simulink model "Trial_Sim_Jonny"  (R2020b)
settings: Solver=VariableStepAuto  StartTime=0.0  StopTime=10.0  RelTol=1e-3
values from neighbouring files (symbols this model uses):
  A_AD = horzcat(A_i, A_ii)    [Trial_Script.m]
  A_kal = [0 0 0 1 0 0 ... (first row only)    [Trial_Script.m]
  B_AD = horzcat(B_i, B_ii)    [Trial_Script.m]
  B_kal = [0 0 0 0 0 0 ... (first row only)    [Trial_Script.m]
  C_AD = eye(6)    [Trial_Script.m]
  C_D = 0.6    [Trial_Script.m]
  C_kal = eye(6)    [Trial_Script.m]
  D_AD = zeros(6)    [Trial_Script.m]
  D_kal = zeros(6)    [Trial_Script.m]
  g = 9.81    [Trial_Script.m]
  I_inv = Inertia_inv    [Trial_Script.m]
  m = 300    [Trial_Script.m]
  pid_Mx = [pid_Mx.Kp, pid_Mx.Ki, pid_Mx.Kd]    [Trial_Script.m]
  pid_My = [pid_My.Kp, pid_My.Ki, pid_My.Kd]    [Trial_Script.m]
  pid_Mz = [pid_Mz.Kp, pid_Mz.Ki, pid_Mz.Kd]    [Trial_Script.m]
  r_0 = [0;0;0]    [Trial_Script.m]
  rho = 1.225    [Trial_Script.m]
  S = 1*1.8    (= 1.8)    [Trial_Script.m]
  T = 10.5    [Trial_Script.m]    (also in temp2.m = readtable('proparms.txt','Delimiter',' '))
  time_delay = 0.1    [Trial_Script.m]
  v_0 = [0;0;0]    [Trial_Script.m]
  w_0 = [0;0;0]    [Trial_Script.m]
undefined symbols (not defined in the file or in its folder): Continuous, Time
libraries: pid_lib x6, ctrlSharedLib x2, simulink x2, dspmtrx3 x1
settings Model: Creator=Jonathan van Zyl  LastModifiedBy=Jonathan van Zyl

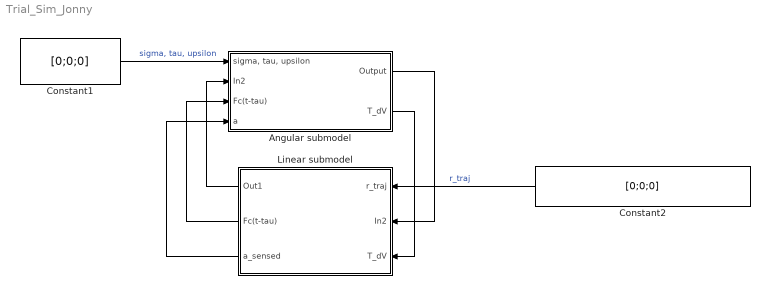
== system Trial_Sim_Jonny ==
  Angular submodel : Subsystem
  Constant1 : Constant  Value=[0;0;0]
  Constant2 : Constant  Value=[0;0;0]
  Linear submodel : Subsystem
  wires:
  Constant1/1 -> Angular submodel/1("sigma, tau, upsilon")  "sigma, tau, upsilon"
  Constant2/1 -> Linear submodel/1(r_traj)  "r_traj"
  Angular submodel/1(Output) -> Linear submodel/2(In2)
  Angular submodel/2(T_dV) -> Linear submodel/3(T_dV)
  Linear submodel/1(Out1) -> Angular submodel/2(In2)
  Linear submodel/2(Fc(t-tau)) -> Angular submodel/3(Fc(t-tau))
  Linear submodel/3(a_sensed) -> Angular submodel/4(a)

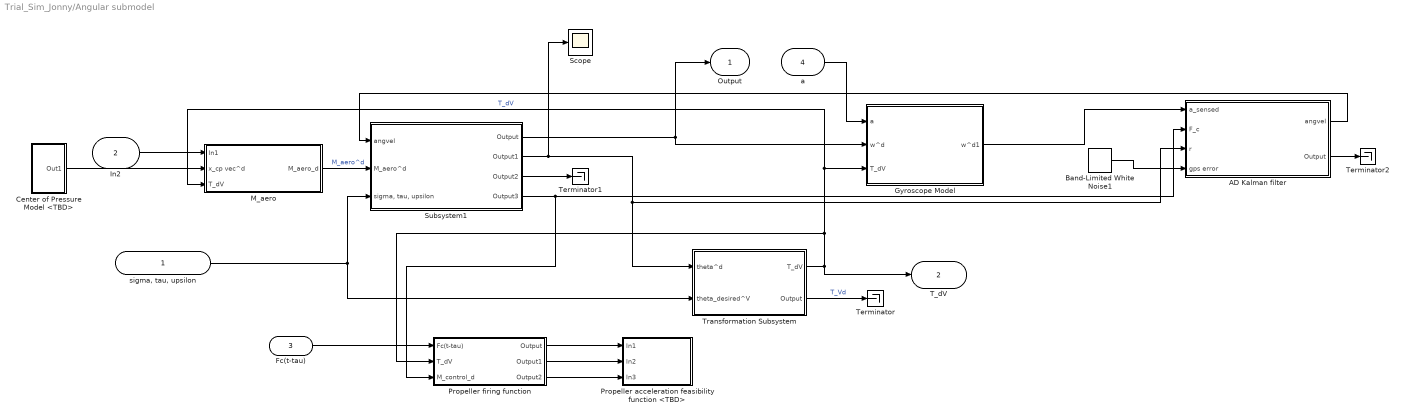
== system Trial_Sim_Jonny/Angular submodel ==
  "sigma, tau, upsilon" : Inport
  In2 : Inport  Port=2
  Fc(t-tau) : Inport  Port=3
  a : Inport  Port=4
  AD Kalman filter : Subsystem
  Band-Limited White Noise1 : simulink/Sources/Band-Limited White Noise  Cov=[0.00001]  Ts=0.1  seed=[23341]
  Center of Pressure Model <TBD> : Subsystem
  Gyroscope Model : Subsystem
  M_aero : Subsystem
  Propeller acceleration feasibility function <TBD> : Subsystem
  Propeller firing function : Subsystem
  Scope : Scope
  Subsystem1 : Subsystem
  Terminator : Terminator
  Terminator1 : Terminator
  Terminator2 : Terminator
  Transformation Subsystem : Subsystem
  Output : Outport
  T_dV : Outport  Port=2
  wires:
  Subsystem1/3(Output2) -> Terminator1/1
  Transformation Subsystem/1(T_dV) -> M_aero/3(T_dV), Gyroscope Model/3(T_dV), Propeller firing function/2(T_dV), T_dV/1  "T_dV"
  Subsystem1/4(Output3) -> Propeller firing function/3(M_control_d), AD Kalman filter/2(F_c)
  Propeller firing function/3(Output2) -> Propeller acceleration feasibility function <TBD>/3(In3)
  Center of Pressure Model <TBD>/1(Out1) -> M_aero/2(x_cp vec^d)
  "sigma, tau, upsilon"/1 -> Transformation Subsystem/2(theta_desired^V), Subsystem1/3("sigma, tau, upsilon")
  AD Kalman filter/1(angvel) -> Subsystem1/1(angvel)
  Propeller firing function/2(Output1) -> Propeller acceleration feasibility function <TBD>/2(In2)
  Subsystem1/2(Output1) -> Scope/1, AD Kalman filter/3(r), Transformation Subsystem/1(theta^d)
  M_aero/1(M_aero_d) -> Subsystem1/2(M_aero^d)  "M_aero^d"
  AD Kalman filter/2(Output) -> Terminator2/1
  Propeller firing function/1(Output) -> Propeller acceleration feasibility function <TBD>/1(In1)
  Transformation Subsystem/2(Output) -> Terminator/1  "T_Vd"
  Gyroscope Model/1(w^d1) -> AD Kalman filter/1(a_sensed)
  Subsystem1/1(Output) -> Output/1, Gyroscope Model/2(w^d)
  Band-Limited White Noise1/1 -> AD Kalman filter/4(gps error)
  a/1 -> Gyroscope Model/1(a)
  Fc(t-tau)/1 -> Propeller firing function/1(Fc(t-tau))
  In2/1 -> M_aero/1(In1)

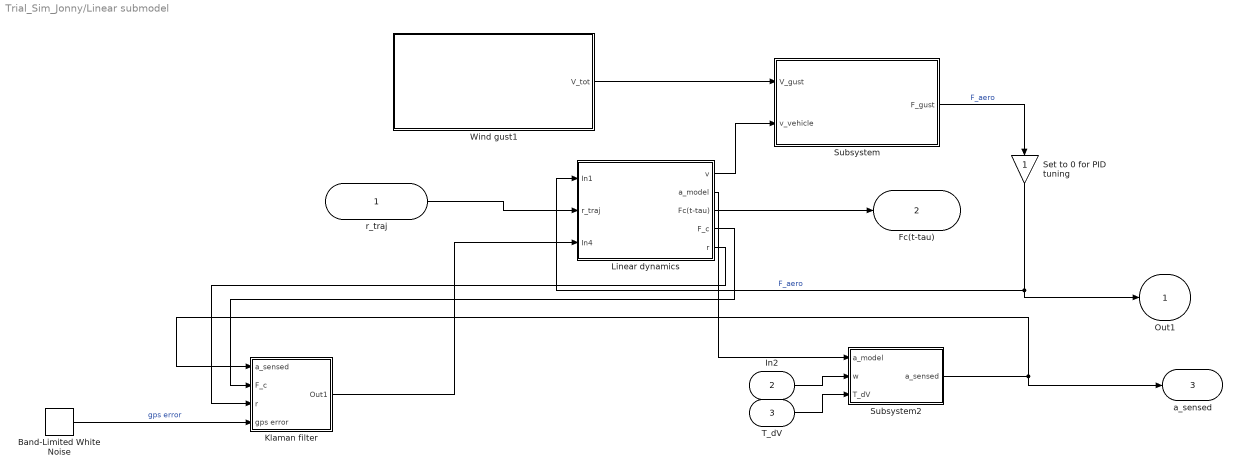
== system Trial_Sim_Jonny/Linear submodel ==
  r_traj : Inport
  In2 : Inport  Port=2
  T_dV : Inport  Port=3
  Band-Limited White Noise : simulink/Sources/Band-Limited White Noise  Cov=[0.00001]  Ts=0.1  seed=[23341]
  Klaman filter : Subsystem
  Linear dynamics : Subsystem
  Set to 0 for PID tuning : Gain
  Subsystem : Subsystem
  Subsystem2 : Subsystem
  Wind gust1 : Subsystem
  Out1 : Outport
  Fc(t-tau) : Outport  Port=2
  a_sensed : Outport  Port=3
  wires:
  Set to 0 for PID tuning/1 -> Out1/1, Linear dynamics/1(In1)  "F_aero"
  Linear dynamics/3(Fc(t-tau)) -> Fc(t-tau)/1
  Wind gust1/1(V_tot) -> Subsystem/1(V_gust)
  Band-Limited White Noise/1 -> Klaman filter/4(gps error)  "gps error"
  Subsystem2/1(a_sensed) -> Klaman filter/1(a_sensed), a_sensed/1
  Subsystem/1(F_gust) -> Set to 0 for PID tuning/1  "F_aero"
  Linear dynamics/1(v) -> Subsystem/2(v_vehicle)
  Klaman filter/1(Out1) -> Linear dynamics/3(In4)
  Linear dynamics/4(F_c) -> Klaman filter/2(F_c)
  Linear dynamics/5(r) -> Klaman filter/3(r)
  Linear dynamics/2(a_model) -> Subsystem2/1(a_model)
  In2/1 -> Subsystem2/2(w)
  T_dV/1 -> Subsystem2/3(T_dV)
  r_traj/1 -> Linear dynamics/2(r_traj)

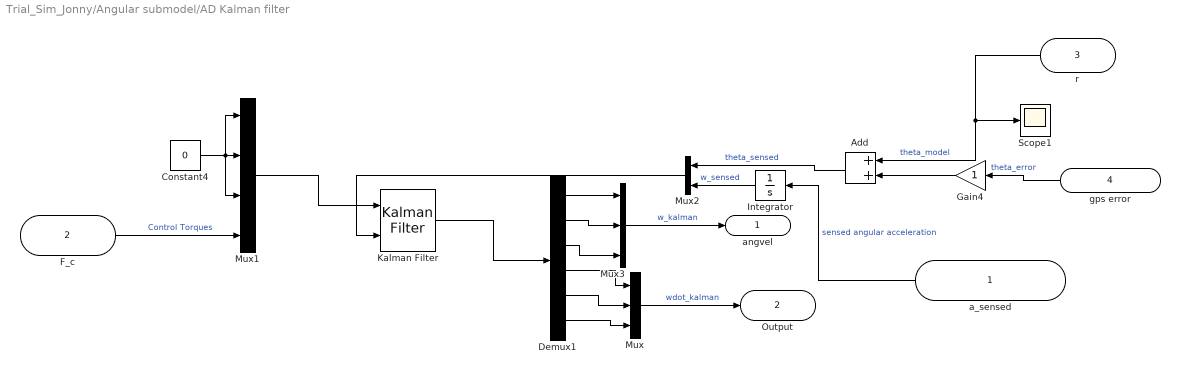
== system Trial_Sim_Jonny/Angular submodel/AD Kalman filter ==
  a_sensed : Inport
  F_c : Inport  Port=2
  r : Inport  Port=3
  gps error : Inport  Port=4
  Add : Sum
  Constant4 : Constant  Value=0
  Demux1 : Demux  Outputs=6
  Gain4 : Gain
  Integrator : Integrator  InitialCondition=w_0
  Kalman Filter : ctrlSharedLib/Kalman Filter  TimeDomain=Continuous-Time  UseCurrentEstimator=on  ModelSource=Individual A, B, C, D matrices  ModelSourceVariable=ss(0.95,1,1,0,1)  A=A_AD  B=B_AD  C=C_AD  D=D_AD  NumberOfStates=1  NumberOfInputs=1  NumberOfOutputs=1  InitialEstimateSource=Dialog  X0=[0;0;0;0;0;0]  P0=10  UseK=off  UseGH=off  NumberOfProcessNoiseInputs=1  G=1  TimeInvariantG=on  H=0  TimeInvariantH=on  Q=0.05  TimeInvariantQ=on  R=1  TimeInvariantR=on  N=0  TimeInvariantN=on  AddInputPort=on  AddEnablePort=off  OutputEstimatedY=off  OutputP=off  Ts=-1
  Mux : Mux  Inputs=3
  Mux1 : Mux
  Mux2 : Mux  Inputs=2
  Mux3 : Mux  Inputs=3
  Scope1 : Scope
  angvel : Outport
  Output : Outport  Port=2
  wires:
  Demux1/5 -> Mux/2
  Mux2/1 -> Kalman Filter/2
  Constant4/1 -> Mux1/3, Mux1/1, Mux1/2
  gps error/1 -> Gain4/1  "theta_error"
  r/1 -> Scope1/1, Add/1  "theta_model"
  Demux1/4 -> Mux/1
  Demux1/2 -> Mux3/2
  Mux1/1 -> Kalman Filter/1
  F_c/1 -> Mux1/4  "Control Torques"
  Demux1/1 -> Mux3/1
  Kalman Filter/1 -> Demux1/1
  Demux1/6 -> Mux/3
  Gain4/1 -> Add/2
  Demux1/3 -> Mux3/3
  Integrator/1 -> Mux2/2  "w_sensed"
  Add/1 -> Mux2/1  "theta_sensed"
  Mux3/1 -> angvel/1  "w_kalman"
  a_sensed/1 -> Integrator/1  "sensed angular acceleration"
  Mux/1 -> Output/1  "wdot_kalman"

== system Trial_Sim_Jonny/Angular submodel/Center of Pressure Model <TBD> ==
  Constant1 : Constant  Value=[0.1;0.2; 0.05]
  Out1 : Outport
  wires:
  Constant1/1 -> Out1/1  "x_cp"

== system Trial_Sim_Jonny/Angular submodel/Gyroscope Model ==
  a : Inport
  w^d : Inport  Port=2
  T_dV : Inport  Port=3
  Terminator : Terminator
  Terminator1 : Terminator
  w^d1 : Outport
  wires:
  w^d/1 -> w^d1/1
  T_dV/1 -> Terminator/1
  a/1 -> Terminator1/1

== system Trial_Sim_Jonny/Angular submodel/M_aero ==
  In1 : Inport
  x_cp vec^d : Inport  Port=2
  T_dV : Inport  Port=3
  Matrix Multiply : Product  Multiplication=Matrix(*)
  Matrix Multiply1 : Product
  M_aero_d : Outport
  wires:
  Matrix Multiply/1 -> Matrix Multiply1/2  "F_dis^d"
  x_cp vec^d/1 -> Matrix Multiply1/1  "x_cp"
  T_dV/1 -> Matrix Multiply/1
  In1/1 -> Matrix Multiply/2  "F_gust"
  Matrix Multiply1/1 -> M_aero_d/1  "M_aero_d"

== system Trial_Sim_Jonny/Angular submodel/Propeller acceleration feasibility function <TBD> ==
  In1 : Inport
  In2 : Inport  Port=2
  In3 : Inport  Port=3
  Terminator4 : Terminator
  Terminator5 : Terminator
  Terminator6 : Terminator
  wires:
  In1/1 -> Terminator4/1
  In2/1 -> Terminator5/1
  In3/1 -> Terminator6/1

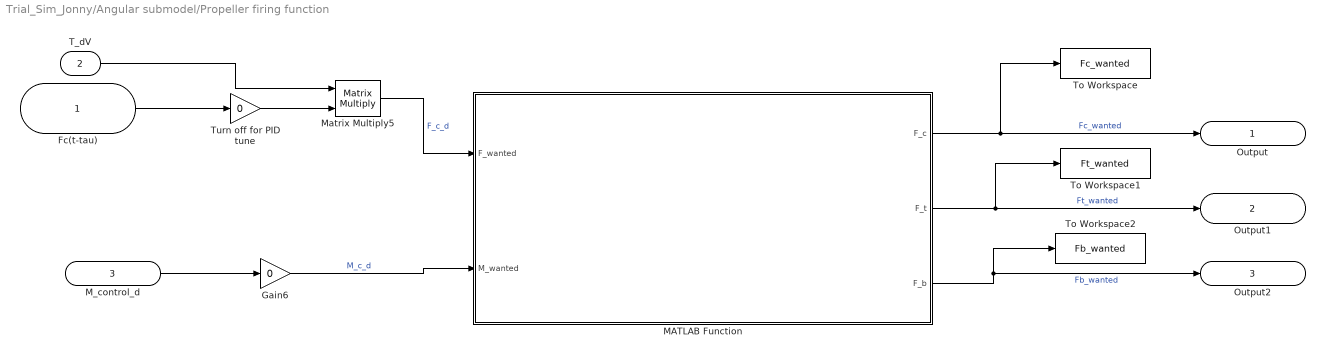
== system Trial_Sim_Jonny/Angular submodel/Propeller firing function ==
  Fc(t-tau) : Inport
  T_dV : Inport  Port=2
  M_control_d : Inport  Port=3
  Gain6 : Gain  Gain=0
  MATLAB Function : MATLAB Function  TreatAsAtomicUnit=on
  Matrix Multiply5 : Product  Multiplication=Matrix(*)
  To Workspace : ToWorkspace  VariableName=Fc_wanted  SaveFormat=Timeseries  SampleTime=-1
  To Workspace1 : ToWorkspace  VariableName=Ft_wanted  SaveFormat=Timeseries  SampleTime=-1
  To Workspace2 : ToWorkspace  VariableName=Fb_wanted  SaveFormat=Timeseries  SampleTime=-1
  Turn off for PID tune : Gain  Gain=0
  Output : Outport
  Output1 : Outport  Port=2
  Output2 : Outport  Port=3
  wires:
  Turn off for PID tune/1 -> Matrix Multiply5/2
  Fc(t-tau)/1 -> Turn off for PID tune/1
  Matrix Multiply5/1 -> MATLAB Function/1(F_wanted)  "F_c_d"
  T_dV/1 -> Matrix Multiply5/1
  M_control_d/1 -> Gain6/1
  Gain6/1 -> MATLAB Function/2(M_wanted)  "M_c_d"
  MATLAB Function/2(F_t) -> To Workspace1/1, Output1/1  "Ft_wanted"
  MATLAB Function/3(F_b) -> Output2/1, To Workspace2/1  "Fb_wanted"
  MATLAB Function/1(F_c) -> To Workspace/1, Output/1  "Fc_wanted"

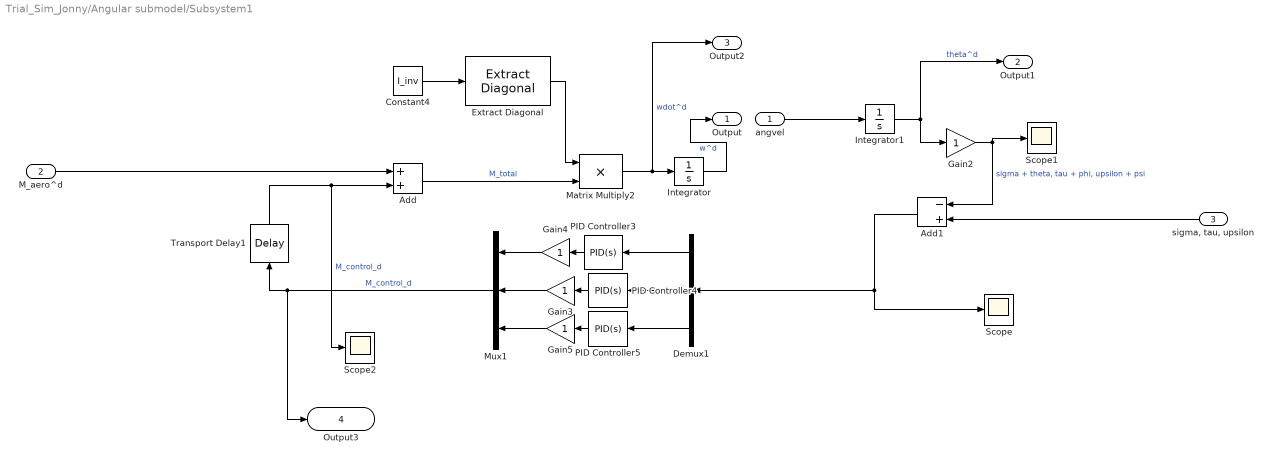
== system Trial_Sim_Jonny/Angular submodel/Subsystem1 ==
  angvel : Inport
  M_aero^d : Inport  Port=2
  "sigma, tau, upsilon" : Inport  Port=3
  Add : Sum
  Add1 : Sum  Inputs=-+
  Constant4 : Constant  Value=I_inv
  Demux1 : Demux  Outputs=3
  Extract Diagonal : dspmtrx3/Extract Diagonal
      settings: SourceProductBaseCode=DS
  Gain{2..5} (4 alike) : Gain
  Integrator : Integrator  InitialCondition=[0;0;0]
  Integrator1 : Integrator  InitialCondition=[0;0;0]
  Matrix Multiply2 : Product
  Mux1 : Mux  Inputs=3
  PID Controller3 : pid_lib/PID Controller  Controller=PID  Form=Parallel  TimeDomain=Continuous-time  UseExternalTs=off  SampleTime=-1  IntegratorMethod=Forward Euler  FilterMethod=Forward Euler  ControllerParametersSource=internal  P=pid_Mx(1)  I=pid_Mx(2)  D=pid_Mx(3)  UseFilter=on  N=546.991859681686  TunerSelectOption=Transfer Function Based (PID Tuner App)  InitialConditionSource=internal  InitialConditionForIntegrator=0  InitialConditionForFilter=0  DifferentiatorICPrevScaledInput=0  ExternalReset=none  TrackingMode=off  Kt=1  LimitOutput=off  SatLimitsSource=internal  UpperSaturationLimit=inf  LowerSaturationLimit=-inf  LinearizeAsGain=on  AntiWindupMode=none  Kb=1  POutMin=[]  POutMax=[]  IOutMin=[]  IOutMax=[]  DOutMin=[]  DOutMax=[]  NOutMin=[]  NOutMax=[]  SumOutMin=[]  SumOutMax=[]  SaturationOutMin=[]  SaturationOutMax=[]  PParamMin=[]  PParamMax=[]  IParamMin=[]  IParamMax=[]  DParamMin=[]  DParamMax=[]  NParamMin=[]  NParamMax=[]  KbParamMin=[]  KbParamMax=[]  KtParamMin=[]  KtParamMax=[]  KbOutMin=[]  KbOutMax=[]  KtOutMin=[]  KtOutMax=[]  IntegratorOutMin=[]  IntegratorOutMax=[]  FilterOutMin=[]  FilterOutMax=[]  SumI1OutMin=[]  SumI1OutMax=[]  SumI2OutMin=[]  SumI2OutMax=[]  SumI3OutMin=[]  SumI3OutMax=[]  SumI4OutMin=[]  SumI4OutMax=[]  SumDOutMin=[]  SumDOutMax=[]  DifferentiatorOutMin=[]  DifferentiatorOutMax=[]  FilterDiffOutCoefMin=[]  FilterDiffOutCoefMax=[]  ReciprocalOutMin=[]  ReciprocalOutMax=[]  SumDenOutMin=[]  SumDenOutMax=[]  SumNumOutMin=[]  SumNumOutMax=[]  DivideOutMin=[]  DivideOutMax=[]  UdiffTsProdOutMin=[]  UdiffTsProdOutMax=[]  NTsProdOutMin=[]  NTsProdOutMax=[]  UintegralTsProdOutMin=[]  UintegralTsProdOutMax=[]  UngainTsProdOutMin=[]  UngainTsProdOutMax=[]  IntegratorContinuousStateAttributes=''  IntegratorStateMustResolveToSignalObject=off  IntegratorRTWStateStorageClass=Auto  FilterContinuousStateAttributes=''  FilterStateMustResolveToSignalObject=off  FilterRTWStateStorageClass=Auto  ParallelPVariant=InternalParameters  IdealPVariant=Disabled  IVariant=InternalParameters  DVariant=InternalParameters  IntegratorVariant=Continuous  SatVariant=Disabled  AWVariant=Passthrough  PCopyVariant=Disabled  TRVariant=Disabled  FdbkBlocksVariant=Forward  IdealPFdbkVariant=Disabled  SatFdbkVariant=Disabled  DerivativeFilterVariant=ContFilter  NVariant=InternalParameters  NCopyVariant=Disabled  FilterICVariant=InternalICsFilter  IntegratorICVariant=InternalICs  ExternalResetVariant=Disabled  TRSumVariant=Passthrough  SumFdbkVariant=Disabled  SumVariant=Sum_PID  TsampFilterVariant=InternalTs  TsampNgainVariant=Passthrough  TsampIntegralVariant=Passthrough  ExternalSaturationOutDataTypeStr=Inherit: Same as second input
  PID Controller4 : pid_lib/PID Controller  Controller=PID  Form=Parallel  TimeDomain=Continuous-time  UseExternalTs=off  SampleTime=-1  IntegratorMethod=Forward Euler  FilterMethod=Forward Euler  ControllerParametersSource=internal  P=pid_My(1)  I=pid_My(2)  D=pid_My(3)  UseFilter=on  N=10.4897155810233  TunerSelectOption=Transfer Function Based (PID Tuner App)  InitialConditionSource=internal  InitialConditionForIntegrator=0  InitialConditionForFilter=0  DifferentiatorICPrevScaledInput=0  ExternalReset=none  TrackingMode=off  Kt=1  LimitOutput=off  SatLimitsSource=internal  UpperSaturationLimit=inf  LowerSaturationLimit=-inf  LinearizeAsGain=on  AntiWindupMode=none  Kb=1  POutMin=[]  POutMax=[]  IOutMin=[]  IOutMax=[]  DOutMin=[]  DOutMax=[]  NOutMin=[]  NOutMax=[]  SumOutMin=[]  SumOutMax=[]  SaturationOutMin=[]  SaturationOutMax=[]  PParamMin=[]  PParamMax=[]  IParamMin=[]  IParamMax=[]  DParamMin=[]  DParamMax=[]  NParamMin=[]  NParamMax=[]  KbParamMin=[]  KbParamMax=[]  KtParamMin=[]  KtParamMax=[]  KbOutMin=[]  KbOutMax=[]  KtOutMin=[]  KtOutMax=[]  IntegratorOutMin=[]  IntegratorOutMax=[]  FilterOutMin=[]  FilterOutMax=[]  SumI1OutMin=[]  SumI1OutMax=[]  SumI2OutMin=[]  SumI2OutMax=[]  SumI3OutMin=[]  SumI3OutMax=[]  SumI4OutMin=[]  SumI4OutMax=[]  SumDOutMin=[]  SumDOutMax=[]  DifferentiatorOutMin=[]  DifferentiatorOutMax=[]  FilterDiffOutCoefMin=[]  FilterDiffOutCoefMax=[]  ReciprocalOutMin=[]  ReciprocalOutMax=[]  SumDenOutMin=[]  SumDenOutMax=[]  SumNumOutMin=[]  SumNumOutMax=[]  DivideOutMin=[]  DivideOutMax=[]  UdiffTsProdOutMin=[]  UdiffTsProdOutMax=[]  NTsProdOutMin=[]  NTsProdOutMax=[]  UintegralTsProdOutMin=[]  UintegralTsProdOutMax=[]  UngainTsProdOutMin=[]  UngainTsProdOutMax=[]  IntegratorContinuousStateAttributes=''  IntegratorStateMustResolveToSignalObject=off  IntegratorRTWStateStorageClass=Auto  FilterContinuousStateAttributes=''  FilterStateMustResolveToSignalObject=off  FilterRTWStateStorageClass=Auto  ParallelPVariant=InternalParameters  IdealPVariant=Disabled  IVariant=InternalParameters  DVariant=InternalParameters  IntegratorVariant=Continuous  SatVariant=Disabled  AWVariant=Passthrough  PCopyVariant=Disabled  TRVariant=Disabled  FdbkBlocksVariant=Forward  IdealPFdbkVariant=Disabled  SatFdbkVariant=Disabled  DerivativeFilterVariant=ContFilter  NVariant=InternalParameters  NCopyVariant=Disabled  FilterICVariant=InternalICsFilter  IntegratorICVariant=InternalICs  ExternalResetVariant=Disabled  TRSumVariant=Passthrough  SumFdbkVariant=Disabled  SumVariant=Sum_PID  TsampFilterVariant=InternalTs  TsampNgainVariant=Passthrough  TsampIntegralVariant=Passthrough  ExternalSaturationOutDataTypeStr=Inherit: Same as second input
  PID Controller5 : pid_lib/PID Controller  Controller=PID  Form=Parallel  TimeDomain=Continuous-time  UseExternalTs=off  SampleTime=-1  IntegratorMethod=Forward Euler  FilterMethod=Forward Euler  ControllerParametersSource=internal  P=pid_Mz(1)  I=pid_Mz(2)  D=pid_Mz(3)  UseFilter=on  N=10.4897155810233  TunerSelectOption=Transfer Function Based (PID Tuner App)  InitialConditionSource=internal  InitialConditionForIntegrator=0  InitialConditionForFilter=0  DifferentiatorICPrevScaledInput=0  ExternalReset=none  TrackingMode=off  Kt=1  LimitOutput=off  SatLimitsSource=internal  UpperSaturationLimit=inf  LowerSaturationLimit=-inf  LinearizeAsGain=on  AntiWindupMode=none  Kb=1  POutMin=[]  POutMax=[]  IOutMin=[]  IOutMax=[]  DOutMin=[]  DOutMax=[]  NOutMin=[]  NOutMax=[]  SumOutMin=[]  SumOutMax=[]  SaturationOutMin=[]  SaturationOutMax=[]  PParamMin=[]  PParamMax=[]  IParamMin=[]  IParamMax=[]  DParamMin=[]  DParamMax=[]  NParamMin=[]  NParamMax=[]  KbParamMin=[]  KbParamMax=[]  KtParamMin=[]  KtParamMax=[]  KbOutMin=[]  KbOutMax=[]  KtOutMin=[]  KtOutMax=[]  IntegratorOutMin=[]  IntegratorOutMax=[]  FilterOutMin=[]  FilterOutMax=[]  SumI1OutMin=[]  SumI1OutMax=[]  SumI2OutMin=[]  SumI2OutMax=[]  SumI3OutMin=[]  SumI3OutMax=[]  SumI4OutMin=[]  SumI4OutMax=[]  SumDOutMin=[]  SumDOutMax=[]  DifferentiatorOutMin=[]  DifferentiatorOutMax=[]  FilterDiffOutCoefMin=[]  FilterDiffOutCoefMax=[]  ReciprocalOutMin=[]  ReciprocalOutMax=[]  SumDenOutMin=[]  SumDenOutMax=[]  SumNumOutMin=[]  SumNumOutMax=[]  DivideOutMin=[]  DivideOutMax=[]  UdiffTsProdOutMin=[]  UdiffTsProdOutMax=[]  NTsProdOutMin=[]  NTsProdOutMax=[]  UintegralTsProdOutMin=[]  UintegralTsProdOutMax=[]  UngainTsProdOutMin=[]  UngainTsProdOutMax=[]  IntegratorContinuousStateAttributes=''  IntegratorStateMustResolveToSignalObject=off  IntegratorRTWStateStorageClass=Auto  FilterContinuousStateAttributes=''  FilterStateMustResolveToSignalObject=off  FilterRTWStateStorageClass=Auto  ParallelPVariant=InternalParameters  IdealPVariant=Disabled  IVariant=InternalParameters  DVariant=InternalParameters  IntegratorVariant=Continuous  SatVariant=Disabled  AWVariant=Passthrough  PCopyVariant=Disabled  TRVariant=Disabled  FdbkBlocksVariant=Forward  IdealPFdbkVariant=Disabled  SatFdbkVariant=Disabled  DerivativeFilterVariant=ContFilter  NVariant=InternalParameters  NCopyVariant=Disabled  FilterICVariant=InternalICsFilter  IntegratorICVariant=InternalICs  ExternalResetVariant=Disabled  TRSumVariant=Passthrough  SumFdbkVariant=Disabled  SumVariant=Sum_PID  TsampFilterVariant=InternalTs  TsampNgainVariant=Passthrough  TsampIntegralVariant=Passthrough  ExternalSaturationOutDataTypeStr=Inherit: Same as second input
  Scope : Scope
  Scope1 : Scope
  Scope2 : Scope
  Transport Delay1 : TransportDelay  DelayTime=time_delay  TransDelayFeedthrough=on
  Output : Outport
  Output1 : Outport  Port=2
  Output2 : Outport  Port=3
  Output3 : Outport  Port=4
  wires:
  Gain5/1 -> Mux1/3
  Transport Delay1/1 -> Scope2/1, Add/2  "M_control_d"
  Demux1/2 -> PID Controller4/1
  Demux1/1 -> PID Controller3/1
  Extract Diagonal/1 -> Matrix Multiply2/1
  Demux1/3 -> PID Controller5/1
  Gain2/1 -> Add1/1, Scope1/1  "sigma + theta, tau + phi, upsilon + psi"
  PID Controller4/1 -> Gain3/1
  Add1/1 -> Scope/1, Demux1/1
  PID Controller5/1 -> Gain5/1
  Gain4/1 -> Mux1/1
  M_aero^d/1 -> Add/1
  Constant4/1 -> Extract Diagonal/1
  Matrix Multiply2/1 -> Output2/1, Integrator/1  "wdot^d"
  Add/1 -> Matrix Multiply2/2  "M_total"
  Integrator/1 -> Output/1  "w^d"
  Mux1/1 -> Output3/1, Transport Delay1/1  "M_control_d"
  Gain3/1 -> Mux1/2
  PID Controller3/1 -> Gain4/1
  Integrator1/1 -> Gain2/1, Output1/1  "theta^d"
  "sigma, tau, upsilon"/1 -> Add1/2
  angvel/1 -> Integrator1/1

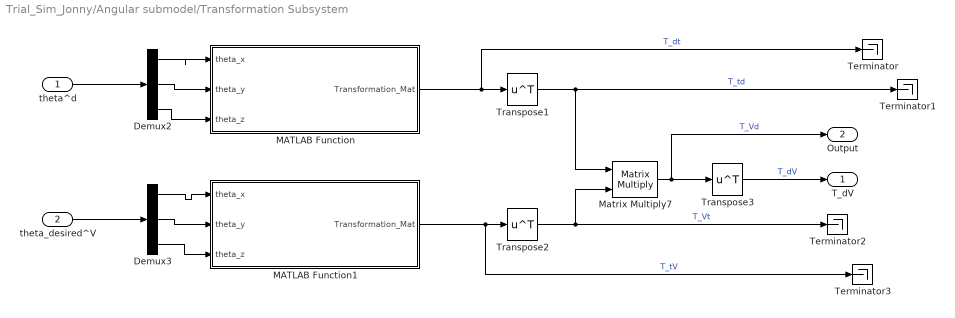
== system Trial_Sim_Jonny/Angular submodel/Transformation Subsystem ==
  theta^d : Inport
  theta_desired^V : Inport  Port=2
  Demux2 : Demux  Outputs=3
  Demux3 : Demux  Outputs=3
  MATLAB Function : MATLAB Function  TreatAsAtomicUnit=on
  MATLAB Function1 : MATLAB Function  TreatAsAtomicUnit=on
  Matrix Multiply7 : Product  Multiplication=Matrix(*)
  Terminator{,1..3} (4 alike) : Terminator
  Transpose1 : Math  Operator=transpose  SaturateOnIntegerOverflow=on
  Transpose2 : Math  Operator=transpose  SaturateOnIntegerOverflow=on
  Transpose3 : Math  Operator=transpose  SaturateOnIntegerOverflow=on
  T_dV : Outport
  Output : Outport  Port=2
  wires:
  Demux3/1 -> MATLAB Function1/1(theta_x)
  Demux2/1 -> MATLAB Function/1(theta_x)
  Transpose2/1 -> Terminator2/1, Matrix Multiply7/2  "T_Vt"
  Demux2/2 -> MATLAB Function/2(theta_y)
  MATLAB Function/1(Transformation_Mat) -> Terminator/1, Transpose1/1  "T_dt"
  Transpose1/1 -> Terminator1/1, Matrix Multiply7/1  "T_td"
  Demux2/3 -> MATLAB Function/3(theta_z)
  MATLAB Function1/1(Transformation_Mat) -> Terminator3/1, Transpose2/1  "T_tV"
  Matrix Multiply7/1 -> Output/1, Transpose3/1  "T_Vd"
  theta_desired^V/1 -> Demux3/1
  Demux3/3 -> MATLAB Function1/3(theta_z)
  Demux3/2 -> MATLAB Function1/2(theta_y)
  Transpose3/1 -> T_dV/1  "T_dV"
  theta^d/1 -> Demux2/1

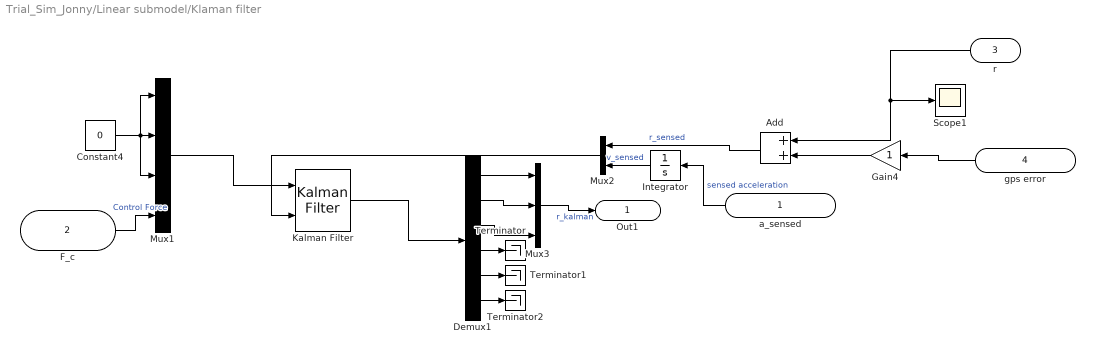
== system Trial_Sim_Jonny/Linear submodel/Klaman filter ==
  a_sensed : Inport
  F_c : Inport  Port=2
  r : Inport  Port=3
  gps error : Inport  Port=4
  Add : Sum
  Constant4 : Constant  Value=0
  Demux1 : Demux  Outputs=6
  Gain4 : Gain
  Integrator : Integrator  InitialCondition=v_0
  Kalman Filter : ctrlSharedLib/Kalman Filter  TimeDomain=Continuous-Time  UseCurrentEstimator=on  ModelSource=Individual A, B, C, D matrices  ModelSourceVariable=ss(0.95,1,1,0,1)  A=A_kal  B=B_kal  C=C_kal  D=D_kal  NumberOfStates=1  NumberOfInputs=1  NumberOfOutputs=1  InitialEstimateSource=Dialog  X0=[0;0;0;0;0;0]  P0=10  UseK=off  UseGH=off  NumberOfProcessNoiseInputs=1  G=1  TimeInvariantG=on  H=0  TimeInvariantH=on  Q=0.05  TimeInvariantQ=on  R=1  TimeInvariantR=on  N=0  TimeInvariantN=on  AddInputPort=on  AddEnablePort=off  OutputEstimatedY=off  OutputP=off  Ts=-1
  Mux1 : Mux
  Mux2 : Mux  Inputs=2
  Mux3 : Mux  Inputs=3
  Scope1 : Scope
  Terminator : Terminator
  Terminator1 : Terminator
  Terminator2 : Terminator
  Out1 : Outport
  wires:
  Demux1/5 -> Terminator1/1
  Mux2/1 -> Kalman Filter/2
  Constant4/1 -> Mux1/3, Mux1/1, Mux1/2
  gps error/1 -> Gain4/1
  r/1 -> Scope1/1, Add/1
  Demux1/4 -> Terminator/1
  Demux1/2 -> Mux3/2
  Mux1/1 -> Kalman Filter/1
  F_c/1 -> Mux1/4  "Control Force"
  Demux1/1 -> Mux3/1
  Kalman Filter/1 -> Demux1/1
  Demux1/6 -> Terminator2/1
  Gain4/1 -> Add/2
  Demux1/3 -> Mux3/3
  Integrator/1 -> Mux2/2  "v_sensed"
  Add/1 -> Mux2/1  "r_sensed"
  Mux3/1 -> Out1/1  "r_kalman"
  a_sensed/1 -> Integrator/1  "sensed acceleration"

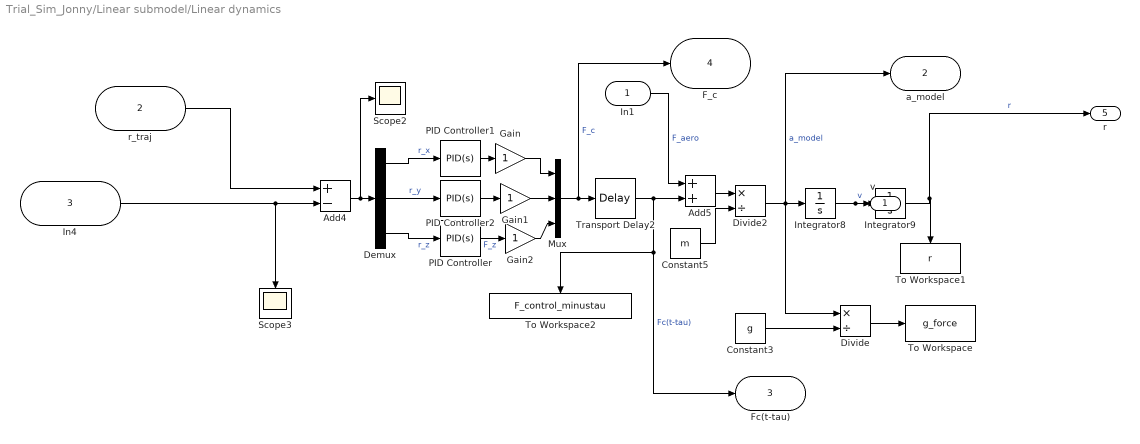
== system Trial_Sim_Jonny/Linear submodel/Linear dynamics ==
  In1 : Inport
  r_traj : Inport  Port=2
  In4 : Inport  Port=3
  Add4 : Sum  Inputs=+-
  Add5 : Sum
  Constant3 : Constant  Value=g
  Constant5 : Constant  Value=m
  Demux : Demux  Outputs=3
  Divide : Product  Inputs=*/
  Divide2 : Product  Inputs=*/
  Gain : Gain
  Gain1 : Gain
  Gain2 : Gain
  Integrator8 : Integrator  InitialCondition=v_0
  Integrator9 : Integrator  InitialCondition=r_0
  Mux : Mux  Inputs=3
  PID Controller : pid_lib/PID Controller  Controller=PID  Form=Parallel  TimeDomain=Continuous-time  UseExternalTs=off  SampleTime=-1  IntegratorMethod=Forward Euler  FilterMethod=Forward Euler  ControllerParametersSource=internal  P=9009.63914578329  I=3464.3602040453  D=5659.73322598295  UseFilter=on  N=27.0214258529072  TunerSelectOption=Transfer Function Based (PID Tuner App)  InitialConditionSource=internal  InitialConditionForIntegrator=0  InitialConditionForFilter=0  DifferentiatorICPrevScaledInput=0  ExternalReset=none  TrackingMode=off  Kt=1  LimitOutput=off  SatLimitsSource=internal  UpperSaturationLimit=inf  LowerSaturationLimit=-inf  LinearizeAsGain=on  AntiWindupMode=none  Kb=1  POutMin=[]  POutMax=[]  IOutMin=[]  IOutMax=[]  DOutMin=[]  DOutMax=[]  NOutMin=[]  NOutMax=[]  SumOutMin=[]  SumOutMax=[]  SaturationOutMin=[]  SaturationOutMax=[]  PParamMin=[]  PParamMax=[]  IParamMin=[]  IParamMax=[]  DParamMin=[]  DParamMax=[]  NParamMin=[]  NParamMax=[]  KbParamMin=[]  KbParamMax=[]  KtParamMin=[]  KtParamMax=[]  KbOutMin=[]  KbOutMax=[]  KtOutMin=[]  KtOutMax=[]  IntegratorOutMin=[]  IntegratorOutMax=[]  FilterOutMin=[]  FilterOutMax=[]  SumI1OutMin=[]  SumI1OutMax=[]  SumI2OutMin=[]  SumI2OutMax=[]  SumI3OutMin=[]  SumI3OutMax=[]  SumI4OutMin=[]  SumI4OutMax=[]  SumDOutMin=[]  SumDOutMax=[]  DifferentiatorOutMin=[]  DifferentiatorOutMax=[]  FilterDiffOutCoefMin=[]  FilterDiffOutCoefMax=[]  ReciprocalOutMin=[]  ReciprocalOutMax=[]  SumDenOutMin=[]  SumDenOutMax=[]  SumNumOutMin=[]  SumNumOutMax=[]  DivideOutMin=[]  DivideOutMax=[]  UdiffTsProdOutMin=[]  UdiffTsProdOutMax=[]  NTsProdOutMin=[]  NTsProdOutMax=[]  UintegralTsProdOutMin=[]  UintegralTsProdOutMax=[]  UngainTsProdOutMin=[]  UngainTsProdOutMax=[]  IntegratorContinuousStateAttributes=''  IntegratorStateMustResolveToSignalObject=off  IntegratorRTWStateStorageClass=Auto  FilterContinuousStateAttributes=''  FilterStateMustResolveToSignalObject=off  FilterRTWStateStorageClass=Auto  ParallelPVariant=InternalParameters  IdealPVariant=Disabled  IVariant=InternalParameters  DVariant=InternalParameters  IntegratorVariant=Continuous  SatVariant=Disabled  AWVariant=Passthrough  PCopyVariant=Disabled  TRVariant=Disabled  FdbkBlocksVariant=Forward  IdealPFdbkVariant=Disabled  SatFdbkVariant=Disabled  DerivativeFilterVariant=ContFilter  NVariant=InternalParameters  NCopyVariant=Disabled  FilterICVariant=InternalICsFilter  IntegratorICVariant=InternalICs  ExternalResetVariant=Disabled  TRSumVariant=Passthrough  SumFdbkVariant=Disabled  SumVariant=Sum_PID  TsampFilterVariant=InternalTs  TsampNgainVariant=Passthrough  TsampIntegralVariant=Passthrough  ExternalSaturationOutDataTypeStr=Inherit: Same as second input
  PID Controller1 : pid_lib/PID Controller  Controller=PID  Form=Parallel  TimeDomain=Continuous-time  UseExternalTs=off  SampleTime=-1  IntegratorMethod=Forward Euler  FilterMethod=Forward Euler  ControllerParametersSource=internal  P=9009.63914576468  I=3464.36020404063  D=5659.73322596604  UseFilter=on  N=27.0214258528983  TunerSelectOption=Transfer Function Based (PID Tuner App)  InitialConditionSource=internal  InitialConditionForIntegrator=0  InitialConditionForFilter=0  DifferentiatorICPrevScaledInput=0  ExternalReset=none  TrackingMode=off  Kt=1  LimitOutput=off  SatLimitsSource=internal  UpperSaturationLimit=inf  LowerSaturationLimit=-inf  LinearizeAsGain=on  AntiWindupMode=none  Kb=1  POutMin=[]  POutMax=[]  IOutMin=[]  IOutMax=[]  DOutMin=[]  DOutMax=[]  NOutMin=[]  NOutMax=[]  SumOutMin=[]  SumOutMax=[]  SaturationOutMin=[]  SaturationOutMax=[]  PParamMin=[]  PParamMax=[]  IParamMin=[]  IParamMax=[]  DParamMin=[]  DParamMax=[]  NParamMin=[]  NParamMax=[]  KbParamMin=[]  KbParamMax=[]  KtParamMin=[]  KtParamMax=[]  KbOutMin=[]  KbOutMax=[]  KtOutMin=[]  KtOutMax=[]  IntegratorOutMin=[]  IntegratorOutMax=[]  FilterOutMin=[]  FilterOutMax=[]  SumI1OutMin=[]  SumI1OutMax=[]  SumI2OutMin=[]  SumI2OutMax=[]  SumI3OutMin=[]  SumI3OutMax=[]  SumI4OutMin=[]  SumI4OutMax=[]  SumDOutMin=[]  SumDOutMax=[]  DifferentiatorOutMin=[]  DifferentiatorOutMax=[]  FilterDiffOutCoefMin=[]  FilterDiffOutCoefMax=[]  ReciprocalOutMin=[]  ReciprocalOutMax=[]  SumDenOutMin=[]  SumDenOutMax=[]  SumNumOutMin=[]  SumNumOutMax=[]  DivideOutMin=[]  DivideOutMax=[]  UdiffTsProdOutMin=[]  UdiffTsProdOutMax=[]  NTsProdOutMin=[]  NTsProdOutMax=[]  UintegralTsProdOutMin=[]  UintegralTsProdOutMax=[]  UngainTsProdOutMin=[]  UngainTsProdOutMax=[]  IntegratorContinuousStateAttributes=''  IntegratorStateMustResolveToSignalObject=off  IntegratorRTWStateStorageClass=Auto  FilterContinuousStateAttributes=''  FilterStateMustResolveToSignalObject=off  FilterRTWStateStorageClass=Auto  ParallelPVariant=InternalParameters  IdealPVariant=Disabled  IVariant=InternalParameters  DVariant=InternalParameters  IntegratorVariant=Continuous  SatVariant=Disabled  AWVariant=Passthrough  PCopyVariant=Disabled  TRVariant=Disabled  FdbkBlocksVariant=Forward  IdealPFdbkVariant=Disabled  SatFdbkVariant=Disabled  DerivativeFilterVariant=ContFilter  NVariant=InternalParameters  NCopyVariant=Disabled  FilterICVariant=InternalICsFilter  IntegratorICVariant=InternalICs  ExternalResetVariant=Disabled  TRSumVariant=Passthrough  SumFdbkVariant=Disabled  SumVariant=Sum_PID  TsampFilterVariant=InternalTs  TsampNgainVariant=Passthrough  TsampIntegralVariant=Passthrough  ExternalSaturationOutDataTypeStr=Inherit: Same as second input
  PID Controller2 : pid_lib/PID Controller  Controller=PID  Form=Parallel  TimeDomain=Continuous-time  UseExternalTs=off  SampleTime=-1  IntegratorMethod=Forward Euler  FilterMethod=Forward Euler  ControllerParametersSource=internal  P=9009.63914561028  I=3464.36020397681  D=5659.73322587286  UseFilter=on  N=27.0214258527793  TunerSelectOption=Transfer Function Based (PID Tuner App)  InitialConditionSource=internal  InitialConditionForIntegrator=0  InitialConditionForFilter=0  DifferentiatorICPrevScaledInput=0  ExternalReset=none  TrackingMode=off  Kt=1  LimitOutput=off  SatLimitsSource=internal  UpperSaturationLimit=inf  LowerSaturationLimit=-inf  LinearizeAsGain=on  AntiWindupMode=none  Kb=1  POutMin=[]  POutMax=[]  IOutMin=[]  IOutMax=[]  DOutMin=[]  DOutMax=[]  NOutMin=[]  NOutMax=[]  SumOutMin=[]  SumOutMax=[]  SaturationOutMin=[]  SaturationOutMax=[]  PParamMin=[]  PParamMax=[]  IParamMin=[]  IParamMax=[]  DParamMin=[]  DParamMax=[]  NParamMin=[]  NParamMax=[]  KbParamMin=[]  KbParamMax=[]  KtParamMin=[]  KtParamMax=[]  KbOutMin=[]  KbOutMax=[]  KtOutMin=[]  KtOutMax=[]  IntegratorOutMin=[]  IntegratorOutMax=[]  FilterOutMin=[]  FilterOutMax=[]  SumI1OutMin=[]  SumI1OutMax=[]  SumI2OutMin=[]  SumI2OutMax=[]  SumI3OutMin=[]  SumI3OutMax=[]  SumI4OutMin=[]  SumI4OutMax=[]  SumDOutMin=[]  SumDOutMax=[]  DifferentiatorOutMin=[]  DifferentiatorOutMax=[]  FilterDiffOutCoefMin=[]  FilterDiffOutCoefMax=[]  ReciprocalOutMin=[]  ReciprocalOutMax=[]  SumDenOutMin=[]  SumDenOutMax=[]  SumNumOutMin=[]  SumNumOutMax=[]  DivideOutMin=[]  DivideOutMax=[]  UdiffTsProdOutMin=[]  UdiffTsProdOutMax=[]  NTsProdOutMin=[]  NTsProdOutMax=[]  UintegralTsProdOutMin=[]  UintegralTsProdOutMax=[]  UngainTsProdOutMin=[]  UngainTsProdOutMax=[]  IntegratorContinuousStateAttributes=''  IntegratorStateMustResolveToSignalObject=off  IntegratorRTWStateStorageClass=Auto  FilterContinuousStateAttributes=''  FilterStateMustResolveToSignalObject=off  FilterRTWStateStorageClass=Auto  ParallelPVariant=InternalParameters  IdealPVariant=Disabled  IVariant=InternalParameters  DVariant=InternalParameters  IntegratorVariant=Continuous  SatVariant=Disabled  AWVariant=Passthrough  PCopyVariant=Disabled  TRVariant=Disabled  FdbkBlocksVariant=Forward  IdealPFdbkVariant=Disabled  SatFdbkVariant=Disabled  DerivativeFilterVariant=ContFilter  NVariant=InternalParameters  NCopyVariant=Disabled  FilterICVariant=InternalICsFilter  IntegratorICVariant=InternalICs  ExternalResetVariant=Disabled  TRSumVariant=Passthrough  SumFdbkVariant=Disabled  SumVariant=Sum_PID  TsampFilterVariant=InternalTs  TsampNgainVariant=Passthrough  TsampIntegralVariant=Passthrough  ExternalSaturationOutDataTypeStr=Inherit: Same as second input
  Scope2 : Scope
  Scope3 : Scope
  To Workspace : ToWorkspace  VariableName=g_force  SaveFormat=Timeseries  SampleTime=-1
      settings: Save2DSignal=2-D array (concatenate along first dimension)
  To Workspace1 : ToWorkspace  VariableName=r  SaveFormat=Timeseries  SampleTime=-1
  To Workspace2 : ToWorkspace  VariableName=F_control_minustau  SaveFormat=Timeseries  SampleTime=-1
  Transport Delay2 : TransportDelay  DelayTime=time_delay  TransDelayFeedthrough=on
  v : Outport
  a_model : Outport  Port=2
  Fc(t-tau) : Outport  Port=3
  F_c : Outport  Port=4
  r : Outport  Port=5
  wires:
  Divide2/1 -> Divide/1, a_model/1, Integrator8/1  "a_model"
  In4/1 -> Add4/2, Scope3/1
  Divide/1 -> To Workspace/1
  r_traj/1 -> Add4/1
  PID Controller2/1 -> Gain1/1
  Add5/1 -> Divide2/1
  Constant5/1 -> Divide2/2
  Demux/1 -> PID Controller1/1  "r_x"
  PID Controller/1 -> Gain2/1  "F_z"
  Gain1/1 -> Mux/2
  Add4/1 -> Scope2/1, Demux/1
  Integrator9/1 -> r/1, To Workspace1/1  "r"
  Demux/2 -> PID Controller2/1  "r_y"
  Transport Delay2/1 -> Fc(t-tau)/1, To Workspace2/1, Add5/2  "Fc(t-tau)"
  PID Controller1/1 -> Gain/1
  Constant3/1 -> Divide/2
  Gain/1 -> Mux/1
  Mux/1 -> F_c/1, Transport Delay2/1  "F_c"
  Demux/3 -> PID Controller/1  "r_z"
  Gain2/1 -> Mux/3
  Integrator8/1 -> Integrator9/1, v/1  "v"
  In1/1 -> Add5/1  "F_aero"

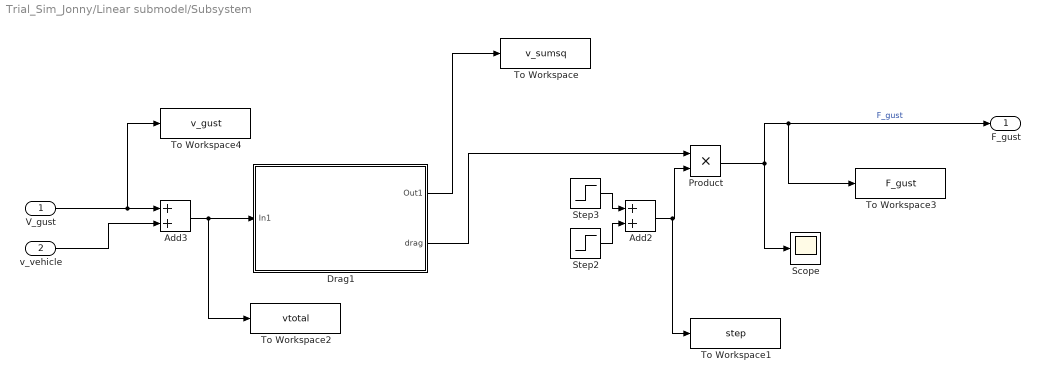
== system Trial_Sim_Jonny/Linear submodel/Subsystem ==
  V_gust : Inport
  v_vehicle : Inport  Port=2
  Add2 : Sum
  Add3 : Sum
  Drag1 : Subsystem
  Product : Product
  Scope : Scope
  Step2 : Step  Time=0  SampleTime=0
  Step3 : Step  Time=10.5  After=-1  SampleTime=0
  To Workspace : ToWorkspace  VariableName=v_sumsq  SampleTime=-1
  To Workspace1 : ToWorkspace  VariableName=step  SaveFormat=Timeseries  SampleTime=-1
  To Workspace2 : ToWorkspace  VariableName=vtotal  SaveFormat=Timeseries  SampleTime=-1
  To Workspace3 : ToWorkspace  VariableName=F_gust  SaveFormat=Timeseries  SampleTime=-1
  To Workspace4 : ToWorkspace  VariableName=v_gust  SaveFormat=Timeseries  SampleTime=-1
  F_gust : Outport
  wires:
  Product/1 -> F_gust/1, To Workspace3/1, Scope/1  "F_gust"
  Step3/1 -> Add2/1
  V_gust/1 -> To Workspace4/1, Add3/1
  Drag1/1(Out1) -> To Workspace/1
  Add3/1 -> Drag1/1(In1), To Workspace2/1
  Add2/1 -> To Workspace1/1, Product/2
  Step2/1 -> Add2/2
  v_vehicle/1 -> Add3/2
  Drag1/2(drag) -> Product/1

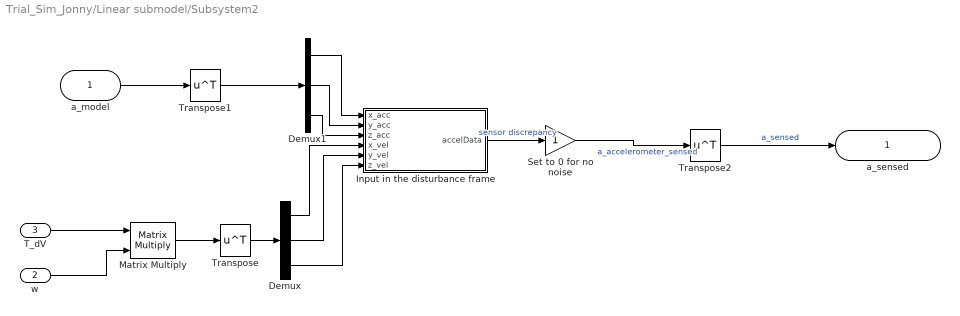
== system Trial_Sim_Jonny/Linear submodel/Subsystem2 ==
  a_model : Inport
  w : Inport  Port=2
  T_dV : Inport  Port=3
  Demux : Demux  Outputs=3
  Demux1 : Demux  Outputs=3
  Input in the disturbance frame : MATLAB Function  TreatAsAtomicUnit=on
  Matrix Multiply : Product  Multiplication=Matrix(*)
  Set to 0 for no noise : Gain
  Transpose : Math  Operator=transpose  SaturateOnIntegerOverflow=on
  Transpose1 : Math  Operator=transpose  SaturateOnIntegerOverflow=on
  Transpose2 : Math  Operator=transpose  SaturateOnIntegerOverflow=on
  a_sensed : Outport
  wires:
  Transpose2/1 -> a_sensed/1  "a_sensed"
  Demux1/1 -> Input in the disturbance frame/1(x_acc)
  Set to 0 for no noise/1 -> Transpose2/1  "a_accelerometer_sensed"
  T_dV/1 -> Matrix Multiply/1
  w/1 -> Matrix Multiply/2
  Demux/1 -> Input in the disturbance frame/4(x_vel)
  a_model/1 -> Transpose1/1
  Input in the disturbance frame/1(accelData) -> Set to 0 for no noise/1  "sensor discrepancy"
  Matrix Multiply/1 -> Transpose/1
  Demux/2 -> Input in the disturbance frame/5(y_vel)
  Demux1/2 -> Input in the disturbance frame/2(y_acc)
  Transpose1/1 -> Demux1/1
  Transpose/1 -> Demux/1
  Demux/3 -> Input in the disturbance frame/6(z_vel)
  Demux1/3 -> Input in the disturbance frame/3(z_acc)

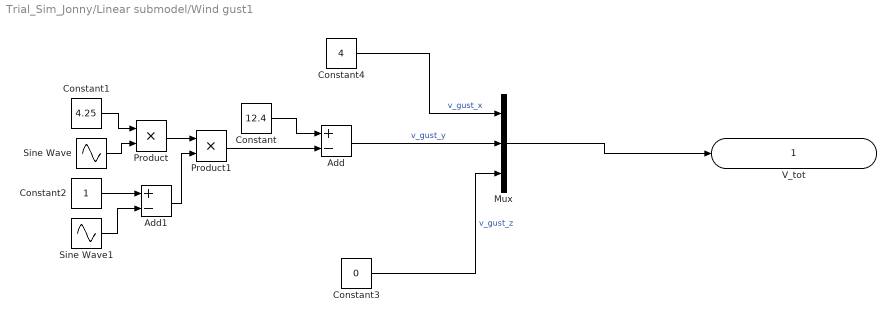
== system Trial_Sim_Jonny/Linear submodel/Wind gust1 ==
  Add : Sum  Inputs=+-
  Add1 : Sum  Inputs=+-
  Constant : Constant  Value=12.4
  Constant1 : Constant  Value=4.25
  Constant2 : Constant
  Constant3 : Constant  Value=0
  Constant4 : Constant  Value=4  VectorParams1D=off
  Mux : Mux  Inputs=3
  Product : Product
  Product1 : Product
  Sine Wave : Sin  Frequency=3*pi/T  SampleTime=0
  Sine Wave1 : Sin  Frequency=2*pi/T  Phase=pi/2  SampleTime=0
  V_tot : Outport
  wires:
  Constant/1 -> Add/1
  Constant1/1 -> Product/1
  Sine Wave/1 -> Product/2
  Constant2/1 -> Add1/1
  Sine Wave1/1 -> Add1/2
  Product/1 -> Product1/1
  Add1/1 -> Product1/2
  Product1/1 -> Add/2
  Add/1 -> Mux/2  "v_gust_y"
  Constant3/1 -> Mux/3  "v_gust_z"
  Mux/1 -> V_tot/1
  Constant4/1 -> Mux/1  "v_gust_x"

== system Trial_Sim_Jonny/Linear submodel/Subsystem/Drag1 ==
  note: Change to C_D and S per side
  In1 : Inport
  Constant1 : Constant  Value=2
  Constant4 : Constant  Value=0.5*rho*C_D*S
  Demux : Demux  Outputs=3
  Mux : Mux  Inputs=3
  Power : Math  Operator=pow  SaturateOnIntegerOverflow=on
  Power1 : Math  Operator=pow  SaturateOnIntegerOverflow=on
  Power2 : Math  Operator=pow  SaturateOnIntegerOverflow=on
  Product1 : Product
  Out1 : Outport
  drag : Outport  Port=2
  wires:
  Constant1/1 -> Power2/2, Power1/2, Power/2
  Power2/1 -> Mux/3
  Power/1 -> Mux/1
  In1/1 -> Demux/1
  Demux/1 -> Power/1
  Demux/3 -> Power2/1
  Demux/2 -> Power1/1
  Power1/1 -> Mux/2
  Constant4/1 -> Product1/2
  Mux/1 -> Out1/1, Product1/1
  Product1/1 -> drag/1  "drag"

== matlab function Trial_Sim_Jonny/Angular submodel/Transformation Subsystem/MATLAB Function ==
  data: theta_x input; Transformation_Mat output; theta_y input; theta_z input
function Transformation_Mat  = Euler(theta_x, theta_y, theta_z)

a = cos(theta_x)*cos(theta_z);
b = cos(theta_x)*sin(theta_z);
c = - sin(theta_x);
d = sin(theta_y)*sin(theta_x)*cos(theta_z) - cos(theta_y)*sin(theta_z);
e = sin(theta_y)*sin(theta_x)*sin(theta_z) + cos(theta_y)*cos(theta_z);
f = sin(theta_y)*cos(theta_x);
g = cos(theta_y)*sin(theta_x)*cos(theta_z) + sin(theta_y)*sin(theta_z);
h = cos(theta_y)*sin(theta_x)*sin(theta_z) - sin(theta_y)*cos(theta_z);
i = cos(theta_y)*cos(theta_x);

Transformation_Mat = [a b c;
    d e f;
    g h i];


end

== matlab function Trial_Sim_Jonny/Angular submodel/Transformation Subsystem/MATLAB Function1 ==
  data: theta_x input; Transformation_Mat output; theta_y input; theta_z input
function Transformation_Mat  = Euler(theta_x, theta_y, theta_z)

a = cos(theta_x)*cos(theta_z);
b = cos(theta_x)*sin(theta_z);
c = - sin(theta_x);
d = sin(theta_y)*sin(theta_x)*cos(theta_z) - cos(theta_y)*sin(theta_z);
e = sin(theta_y)*sin(theta_x)*sin(theta_z) + cos(theta_y)*cos(theta_z);
f = sin(theta_y)*cos(theta_x);
g = cos(theta_y)*sin(theta_x)*cos(theta_z) + sin(theta_y)*sin(theta_z);
h = cos(theta_y)*sin(theta_x)*sin(theta_z) - sin(theta_y)*cos(theta_z);
i = cos(theta_y)*cos(theta_x);

Transformation_Mat = [a b c;
    d e f;
    g h i];


end

== matlab function Trial_Sim_Jonny/Angular submodel/Propeller firing function/MATLAB Function ==
  data: F_wanted input; F_c output; M_wanted input; F_t output; F_b output
function [F_c, F_t, F_b] = propeller_required_forces_control(F_wanted, M_wanted)

%% Load propeller arms data
xc_1 = 0.1;
yc_1 = 0.05;
zc_1 = -0.3;
xc_2 = 0.1;
yc_2 = -0.2;
zc_2 = 0.3;
xc_3 = 0.1;
yc_3 = -0.2;
zc_3 = 0.3;

xt_1 = 0;
yt_1 = -0.9;
zt_1 = 2.4;
xt_2 = 0;
yt_2 = -0.9;
zt_2 = 1.8;
xt_3 = 0;
yt_3 = -0.9;
zt_3 = -1.2;
xt_4 = 0;
yt_4 = -0.9;
zt_4 = -1.2;

xb_1 = -0.01;
yb_1 = 0;
zb_1 = 1.4;
xb_2 = -0.01;
yb_2 = 0;
zb_2 = 1.4;
xb_3 = -0.01;
yb_3 = 0;
zb_3 = 1.4;
xb_4 = -0.01;
yb_4 = 0;
zb_4 = 1.4;
xb_5 = -0.01;
yb_5 = 0;
zb_5 = 1.4;
xb_6 = -0.01;
yb_6 = 0;
zb_6 = 1.4;
%% Decompose force and moment input

F_x = F_wanted(1);
F_y = F_wanted(2);
F_z = F_wanted(3);

M_x = M_wanted(1);
M_y = M_wanted(2);
M_z = M_wanted(3);

%% Find control forces

F_c3 = 2*(M_x + M_y + F_y)/(-yc_1 + zc_1 - yc_2 + zc_2 - 2*yc_3 + 2*zc_3);
F_c2 = F_c3/2;
F_c1 = F_c2;

%% Find top and bottom forces

F_t1 = 1/10 * F_z + M_y/6*(xt_1 + xt_2 + xt_3 + xt_4 + xb_1 + xb_2 + xb_5 + xb_6);
F_t2 = F_t1;
F_t3 = F_t1;
F_t4 = F_t1;
F_b1 = F_t1;
F_b2 = F_t1;
F_b5 = F_t1;
F_b6 = F_t1;

F_b3 = 1/10 * F_z;
F_b4 = F_b3;


%% Make matrix
F_c = [F_c1; F_c2; F_c3];
F_t = [F_t1; F_t2; F_t3; F_t4];
F_b = [F_b1; F_b2; F_b3; F_b4; F_b5; F_b6];

end

== matlab function Trial_Sim_Jonny/Linear submodel/Subsystem2/Input in the disturbance frame ==
  settings: updateMethod=DISCRETE
  data: x_acc input; accelData output; y_acc input; z_acc input; x_vel input; y_vel input; z_vel input
function accelData  = accelerometer(x_acc, y_acc, z_acc, x_vel, y_vel, z_vel)
    %% Outputs: translational acceleration
    %
    % Create gyroscope sensor object
    params = accelparams
    
    acc = [x_acc, y_acc, z_acc];
    angvel = [x_vel, y_vel, z_vel];
    
    % Parameters for simulated signal
    N = 1;       % Number of samples
    Fs = 100;       % Sampling rate
    Fc = 0.25;      % Sinusoidal frequency
    
    
    % Create arrays
    t = (0:(1/Fs):((N-1)/Fs)).';
    acc = acc;          %Input accelerations
    orient = quaternion.ones(N, 1);
    angvel = angvel;
    
    % Generate acceleration data
    imu = imuSensor('SampleRate', Fs, 'Accelerometer', params);
    imu.Accelerometer.MeasurementRange = 100;   % Maximum acceleration accelerometer can measure
    imu.Accelerometer.Resolution = 1/Fs;           % Step size of digital measurements
    
    % Biases
    imu.Accelerometer.BiasInstability = 7.5 / 1000;
    imu.Accelerometer.NoiseDensity = 150 / 1000 / 1000;
    imu.Accelerometer.TemperatureBias = 50 / 1000 / 1000;
    
    
    imu = imuSensor('SampleRate', Fs, 'Accelerometer', params);
    
    accelData = imu(acc, angvel, orient);
    
    accelData(:,3) = accelData(:,3) - 9.81;
    
    accelData(:,1) = accelData(:,1) * -1;
    accelData(:,2) = accelData(:,2) * -1;
    accelData(:,3) = accelData(:,3) * -1;

end
